simulink model "lab3_s"  (R2013b)
settings: Solver=ode45  SolverMode=SingleTasking  StartTime=0.0  StopTime=t_max  MaxStep=0.1  RelTol=1e-3
undefined symbols (not defined in the file): k, k2, Lo, Mo, t0, y0
settings Model: CovMetricSettings=dwe  CovHtmlReporting=off  covSaveCumulativeToWorkspaceVar=off  CovSaveSingleToWorkspaceVar=off  CovExternalEMLEnable=on  Creator=lev  LastModifiedBy=lev
settings DataIOCC: LimitDataPoints=off  SaveFormat=StructureWithTime
settings DebuggingCC: UnderspecifiedInitializationDetection=Simplified  MergeDetectMultiDrivingBlocksExec=error  SolverPrmCheckMsg=none  FrameProcessingCompatibilityMsg=error  SFUnexpectedBacktrackingDiag=error  SFNoUnconditionalDefaultTransitionDiag=error
settings HardwareCC: ProdBitPerPointer=64  ProdLargestAtomicFloat=Float  ProdIntDivRoundTo=Zero  ProdEndianess=LittleEndian  ProdHWDeviceType=Specified
settings ModelReferenceCC: PropagateSignalLabelsOutOfModel=on
settings SFSimCC: SimUseLocalCustomCode=on
settings RTWCC: RTWUseLocalCustomCode=on
settings GRTTargetCC: CodeReplacementLibrary=C99 (ISO)  GeneratePreprocessorConditionals=Use local settings

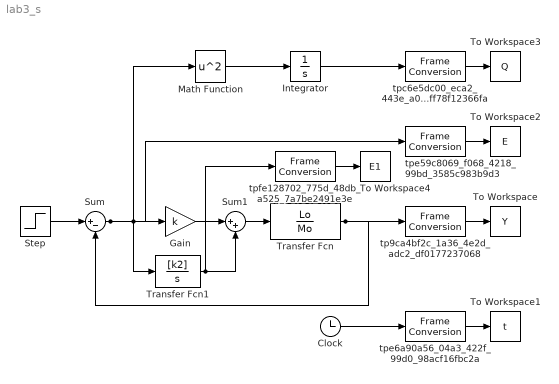
== system lab3_s ==
  Clock : Clock
  Gain : Gain  Gain=k
  Integrator : Integrator
  Math Function : Math  Operator=square  SaturateOnIntegerOverflow=on
  Step : Step  Time=t0  After=y0  SampleTime=0
  Sum : Sum  Inputs=|+-
  Sum1 : Sum  Inputs=|++
  To Workspace : ToWorkspace  VariableName=Y  SampleTime=-1
  To Workspace1 : ToWorkspace  VariableName=t  SampleTime=-1
  To Workspace2 : ToWorkspace  VariableName=E  SampleTime=-1
  To Workspace3 : ToWorkspace  VariableName=Q  SampleTime=-1
  To Workspace4 : ToWorkspace  VariableName=E1  SampleTime=-1
  Transfer Fcn : TransferFcn  Numerator=Lo  Denominator=Mo
  Transfer Fcn1 : TransferFcn  Numerator=[k2]  Denominator=[1 0]
  tp9ca4bf2c_1a36_4e2d_adc2_df0177237068 : FrameConversion  OutFrame=Sample-based
  tpc6e5dc00_eca2_443e_a053_ff78f12366fa : FrameConversion  OutFrame=Sample-based
  tpe59c8069_f068_4218_99bd_3585c983b9d3 : FrameConversion  OutFrame=Sample-based
  tpe6a90a56_04a3_422f_99d0_98acf16fbc2a : FrameConversion  OutFrame=Sample-based
  tpfe128702_775d_48db_a525_7a7be2491e3e : FrameConversion  OutFrame=Sample-based
  wires:
  Transfer Fcn/1 -> Sum/2, tp9ca4bf2c_1a36_4e2d_adc2_df0177237068/1
  Sum/1 -> Transfer Fcn1/1, Gain/1, Math Function/1, tpe59c8069_f068_4218_99bd_3585c983b9d3/1
  Step/1 -> Sum/1
  Sum1/1 -> Transfer Fcn/1
  Transfer Fcn1/1 -> Sum1/2, tpfe128702_775d_48db_a525_7a7be2491e3e/1
  Gain/1 -> Sum1/1
  Math Function/1 -> Integrator/1
  tp9ca4bf2c_1a36_4e2d_adc2_df0177237068/1 -> To Workspace/1
  Clock/1 -> tpe6a90a56_04a3_422f_99d0_98acf16fbc2a/1
  tpe6a90a56_04a3_422f_99d0_98acf16fbc2a/1 -> To Workspace1/1
  tpe59c8069_f068_4218_99bd_3585c983b9d3/1 -> To Workspace2/1
  Integrator/1 -> tpc6e5dc00_eca2_443e_a053_ff78f12366fa/1
  tpc6e5dc00_eca2_443e_a053_ff78f12366fa/1 -> To Workspace3/1
  tpfe128702_775d_48db_a525_7a7be2491e3e/1 -> To Workspace4/1
